simulink model "active_power_and_frequency_delay"  (R2022b)
settings: Solver=VariableStepAuto  StartTime=0.0  StopTime=250.0  RelTol=1e-3
settings Model: Creator=Fabian  LastModifiedBy=Fabian

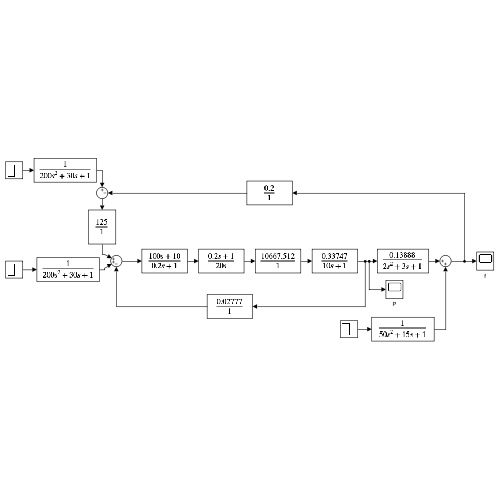
[thumbnail: Simulink's stored preview of the top-level diagram]
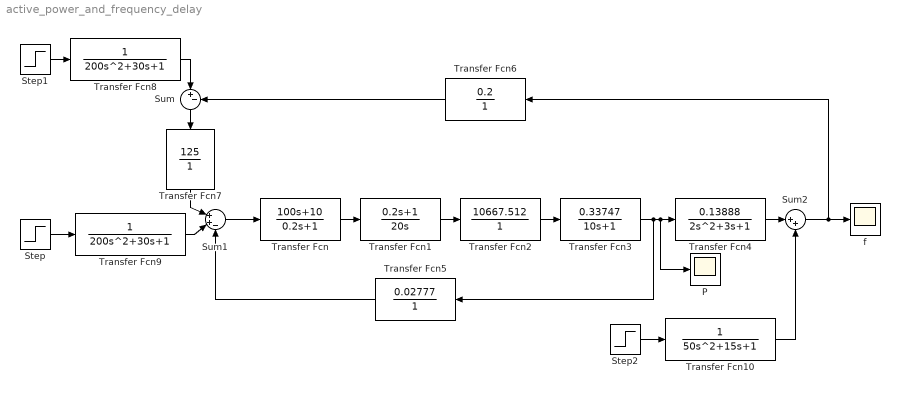
== system active_power_and_frequency_delay ==
  P : Scope
  Step : Step  Time=0  After=10  SampleTime=0
  Step1 : Step  Time=0  After=10  SampleTime=0
  Step2 : Step  Time=150  After=-5  SampleTime=0
  Sum : Sum  Inputs=|+-
  Sum1 : Sum  Inputs=|++-
  Sum2 : Sum  Inputs=|++
  Transfer Fcn : TransferFcn  Numerator=[100 10]  Denominator=[0.2 1]
  Transfer Fcn1 : TransferFcn  Numerator=[0.2 1]  Denominator=[20 0]
  Transfer Fcn10 : TransferFcn  Denominator=[50 15 1]
  Transfer Fcn2 : TransferFcn  Numerator=[10667.512]  Denominator=[1]
  Transfer Fcn3 : TransferFcn  Numerator=[0.33747]  Denominator=[10 1]
  Transfer Fcn4 : TransferFcn  Numerator=[0.13888]  Denominator=[2 3 1]
  Transfer Fcn5 : TransferFcn  Numerator=[0.02777]  Denominator=[1]
  Transfer Fcn6 : TransferFcn  Numerator=[0.2]  Denominator=[1]
  Transfer Fcn7 : TransferFcn  Numerator=[125]  Denominator=[1]
  Transfer Fcn8 : TransferFcn  Denominator=[200 30 1]
  Transfer Fcn9 : TransferFcn  Denominator=[200 30 1]
  f : Scope
  wires:
  Transfer Fcn3/1 -> P/1, Transfer Fcn4/1, Transfer Fcn5/1
  Sum/1 -> Transfer Fcn7/1
  Transfer Fcn7/1 -> Sum1/1
  Transfer Fcn2/1 -> Transfer Fcn3/1
  Sum1/1 -> Transfer Fcn/1
  Transfer Fcn1/1 -> Transfer Fcn2/1
  Transfer Fcn/1 -> Transfer Fcn1/1
  Sum2/1 -> Transfer Fcn6/1, f/1
  Transfer Fcn4/1 -> Sum2/1
  Transfer Fcn5/1 -> Sum1/3
  Transfer Fcn6/1 -> Sum/2
  Step/1 -> Transfer Fcn9/1
  Transfer Fcn9/1 -> Sum1/2
  Step1/1 -> Transfer Fcn8/1
  Transfer Fcn8/1 -> Sum/1
  Step2/1 -> Transfer Fcn10/1
  Transfer Fcn10/1 -> Sum2/2
